simulink model "Battery_switchingR0"  (R2020b)
settings: Solver=FixedStepDiscrete  StartTime=0.0  StopTime=runTime  FixedStep=stepSize
values from neighbouring files (symbols this model uses):
  I1_init = 0    [Battery_run_switchingR0.m]
  I2_init = 0    [Battery_run_switchingR0.m]
  I3_init = 0    [Battery_run_switchingR0.m]
  OCV = param.OCV_init    [Battery_run_switchingR0.m]    (also in Pulse_Test_Process.m = param(8))
  Q = abs(meas_t.Ah(end)-meas_t.Ah(1))    [Battery_run_switchingR0.m]    (also in Parameterization_run_switchingR0.m = abs(meas_optim.Ah(end)-meas_optim.Ah(1)); Pulse_Test_InitialGuess.m = -meas.Ah(end); Pulse_Test_Process.m = Batt.Q*3600)
  R0 = [param.R0_init param.R0_init_chg]    [Battery_run_switchingR0.m]    (also in Pulse_Test_Process.m = param(1))
  R1 = param.R1_init    [Battery_run_switchingR0.m]    (also in Pulse_Test_Process.m = param(2))
  R2 = param.R2_init    [Battery_run_switchingR0.m]    (also in Pulse_Test_Process.m = param(3))
  R3 = param.R3_init    [Battery_run_switchingR0.m]    (also in Pulse_Test_Process.m = param(4))
  SOC = param.SOC    [Battery_run_switchingR0.m]    (also in Parameterization_run_switchingR0.m; Pulse_Test_Process.m = [SOC; oSOC])
  SOC_init = meas_t.SOC(1)    [Battery_run_switchingR0.m]
  tau1 = param.tau1_init    [Battery_run_switchingR0.m]    (also in Pulse_Test_Process.m = param(5))
  tau2 = param.tau2_init    [Battery_run_switchingR0.m]    (also in Pulse_Test_Process.m = param(6))
  tau3 = param.tau3_init    [Battery_run_switchingR0.m]    (also in Pulse_Test_Process.m = param(7))
  useOCVpolynomial = 1    [Battery_run_switchingR0.m]    (also in Parameterization_run_switchingR0.m = 0)
undefined symbols (not defined in the file or in its folder): coeff
settings Model: PacingRate=1000  OrderedModelArguments=off  Creator=Wenlin  LastModifiedBy=Wenlin
settings DataIOCC: OutputOption=AdditionalOutputTimes  OutputTimes=SDO_OutputTimes  ReturnWorkspaceOutputsName=SDOSimTest_Log
settings DebuggingCC: UnderSpecifiedDimensionMsg=warning

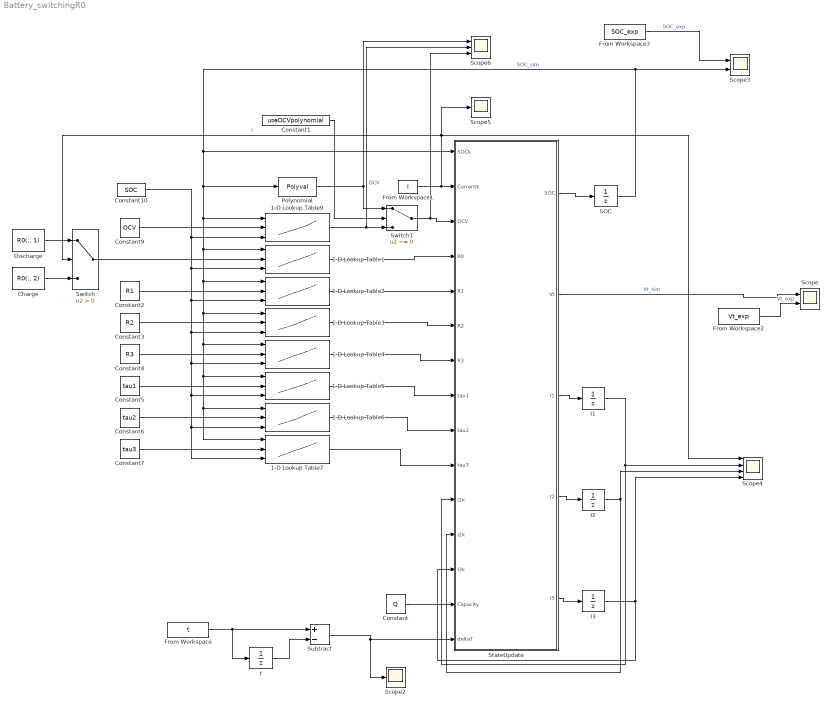
== system Battery_switchingR0 ==
  1-D Lookup Table{1..7,9} (8 alike) : Lookup_n-D  NumberOfTableDimensions=1  BreakpointsForDimension1Source=Input port  BreakpointsForDimension1=SOC  TableSource=Input port  Table=OCV  ExtrapMethod=Clip  UseLastTableValue=on  InternalRulePriority=Speed  RndMeth=Simplest  InputSameDT=on
      settings: InputPortMap=u0,p221,p5
  Charge : Constant  Value=R0(:, 2)
  Constant : Constant  Value=Q
  Constant1 : Constant  Value=useOCVpolynomial
  Constant10 : Constant  Value=SOC
  Constant2 : Constant  Value=R1
  Constant3 : Constant  Value=R2
  Constant4 : Constant  Value=R3
  Constant5 : Constant  Value=tau1
  Constant6 : Constant  Value=tau2
  Constant7 : Constant  Value=tau3
  Constant9 : Constant  Value=OCV
  Discharge : Constant  Value=R0(:, 1)
  From Workspace : FromWorkspace  VariableName=t  OutputAfterFinalValue=Setting to zero
  From Workspace1 : FromWorkspace  VariableName=I
  From Workspace2 : FromWorkspace  VariableName=Vt_exp
  From Workspace3 : FromWorkspace  VariableName=SOC_exp
  I1 : UnitDelay  InitialCondition=I1_init  SampleTime=-1  HasFrameUpgradeWarning=on
  I2 : UnitDelay  InitialCondition=I2_init  SampleTime=-1  HasFrameUpgradeWarning=on
  I3 : UnitDelay  InitialCondition=I3_init  SampleTime=-1  HasFrameUpgradeWarning=on
  Polynomial : Polyval  Coefs=coeff
  SOC : UnitDelay  InitialCondition=SOC_init  SampleTime=-1  HasFrameUpgradeWarning=on
  Scope : Scope  NumInputPorts=2
  Scope2 : Scope
  Scope3 : Scope  NumInputPorts=2
  Scope4 : Scope  NumInputPorts=4
  Scope5 : Scope
  Scope6 : Scope  NumInputPorts=3
  StateUpdate : MATLAB Function  TreatAsAtomicUnit=on
  Subtract : Sum  Inputs=+-
  Switch : Switch  Criteria=u2 > Threshold
  Switch1 : Switch  Criteria=u2 ~= 0
  t : UnitDelay  SampleTime=-1  HasFrameUpgradeWarning=on
  wires:
  Constant6/1 -> 1-D Lookup Table6/2
  StateUpdate/1(SOC) -> SOC/1
  Constant7/1 -> 1-D Lookup Table7/2
  I2/1 -> Scope4/3, StateUpdate/12(I2k)
  Constant4/1 -> 1-D Lookup Table4/2
  StateUpdate/4(I2) -> I2/1
  Constant5/1 -> 1-D Lookup Table5/2
  1-D Lookup Table6/1 -> StateUpdate/9(tau2)
  Constant/1 -> StateUpdate/14(Capacity)
  1-D Lookup Table1/1 -> StateUpdate/4(R0)
  Constant2/1 -> 1-D Lookup Table2/2
  1-D Lookup Table2/1 -> StateUpdate/5(R1)
  From Workspace/1 -> t/1, Subtract/1
  Switch/1 -> 1-D Lookup Table1/2
  I1/1 -> StateUpdate/11(I1k), Scope4/2
  1-D Lookup Table4/1 -> StateUpdate/7(R3)
  Constant10/1 -> 1-D Lookup Table9/3, 1-D Lookup Table3/3, 1-D Lookup Table4/3, 1-D Lookup Table5/3, 1-D Lookup Table7/3, 1-D Lookup Table6/3, 1-D Lookup Table2/3, 1-D Lookup Table1/3
  StateUpdate/2(Vt) -> Scope/1  "Vt_sim"
  Subtract/1 -> Scope2/1, StateUpdate/15(deltaT)
  1-D Lookup Table9/1 -> Scope6/2, Switch1/3  "OCV"
  StateUpdate/3(I1) -> I1/1
  t/1 -> Subtract/2
  From Workspace1/1 -> Scope4/1, Scope5/1, Switch/2, StateUpdate/2(Currentk)  "I"
  SOC/1 -> Polynomial/1, 1-D Lookup Table1/1, 1-D Lookup Table3/1, 1-D Lookup Table4/1, 1-D Lookup Table5/1, 1-D Lookup Table7/1, 1-D Lookup Table6/1, 1-D Lookup Table2/1, 1-D Lookup Table9/1, StateUpdate/1(SOCk), Scope3/2  "SOC_sim"
  StateUpdate/5(I3) -> I3/1
  1-D Lookup Table3/1 -> StateUpdate/6(R2)
  Constant3/1 -> 1-D Lookup Table3/2
  1-D Lookup Table5/1 -> StateUpdate/8(tau1)
  1-D Lookup Table7/1 -> StateUpdate/10(tau3)
  I3/1 -> Scope4/4, StateUpdate/13(I3k)
  From Workspace2/1 -> Scope/2  "Vt_exp"
  From Workspace3/1 -> Scope3/1  "SOC_exp"
  Constant9/1 -> 1-D Lookup Table9/2
  Discharge/1 -> Switch/1
  Charge/1 -> Switch/3
  Switch1/1 -> Scope6/3, StateUpdate/3(OCV)
  Polynomial/1 -> Switch1/1, Scope6/1
  Constant1/1 -> Switch1/2

== matlab function Battery_switchingR0/StateUpdate ==
  data: SOC output; SOCk input; Currentk input; OCV input; R0 input; R1 input; R2 input; R3 input; tau1 input; tau2 input; tau3 input; I1k input; I2k input; I3k input; Capacity input; deltaT input; Vt output; I1 output; I2 output; I3 output
function [SOC, Vt, I1, I2, I3] = StateUpdate(SOCk, Currentk, OCV, R0, R1, R2, R3, tau1, tau2, tau3, I1k, I2k, I3k, Capacity, deltaT)

    Q = Capacity*3600;
    
    % Calculate currents
    I1 =  ( 1 - exp(-deltaT/tau1) ) * Currentk + exp(-deltaT/tau1) * I1k;
    I2 =  ( 1 - exp(-deltaT/tau2) ) * Currentk + exp(-deltaT/tau2) * I2k;
    I3 =  ( 1 - exp(-deltaT/tau3) ) * Currentk + exp(-deltaT/tau3) * I3k;

    % Update voltage & SOC
    Vt   = OCV - (R0*Currentk) - R1*I1 - R2*I2 - R3*I3;
    SOC  = SOCk - (deltaT/Q) * Currentk;

end
